simulink library "magField_reduced_lib"  (R2018b)
settings: Solver=VariableStepAuto  StartTime=0.0  StopTime=10.0  RelTol=1e-3
undefined symbols (not defined in the file or in its folder): fswParams, magField_lib, simParams
libraries: simulink_extras x2, aerolibgravity2 x1
settings Model: Creator=colem  LastModifiedBy=colem

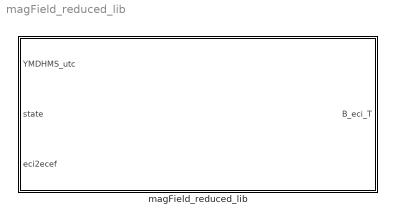
== system magField_reduced_lib ==
  magField_reduced_lib : Subsystem  AncestorBlock=magField_lib/magField_lib

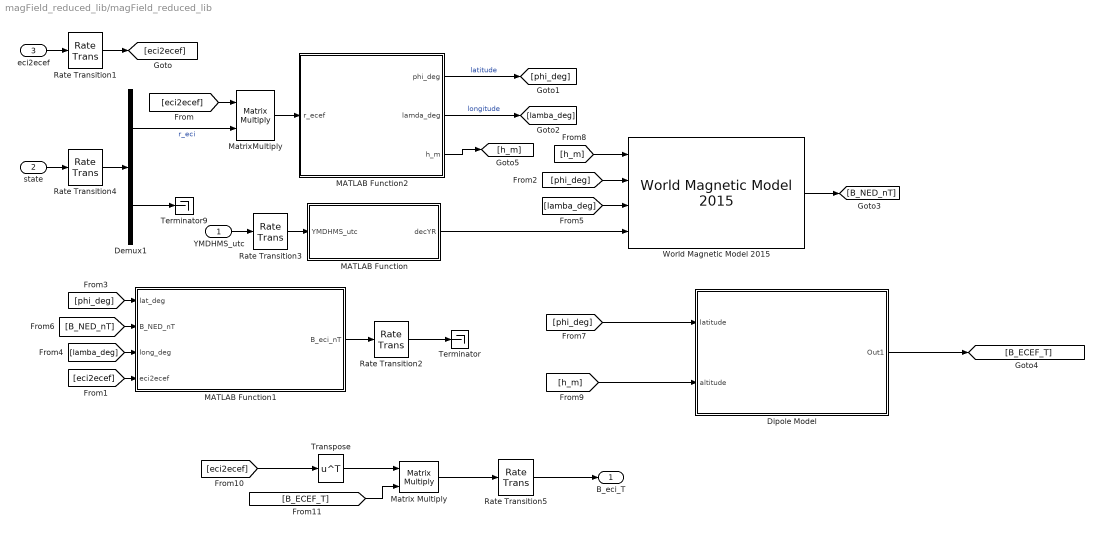
== system magField_reduced_lib/magField_reduced_lib ==
  YMDHMS_utc : Inport
  state : Inport  Port=2
  eci2ecef : Inport  Port=3
  Demux1 : Demux  Outputs=[3 10]
  Dipole Model : Subsystem
  MATLAB Function : MATLAB Function  TreatAsAtomicUnit=on
  MATLAB Function1 : MATLAB Function  TreatAsAtomicUnit=on
  MATLAB Function2 : MATLAB Function  TreatAsAtomicUnit=on
  Matrix Multiply : Product  Multiplication=Matrix(*)
  MatrixMultiply : Product  Multiplication=Matrix(*)
  Rate Transition1 : RateTransition  OutPortSampleTime=simParams.magField.sample_time_s
  Rate Transition2 : RateTransition
  Rate Transition3 : RateTransition  OutPortSampleTime=simParams.magField.sample_time_s
  Rate Transition4 : RateTransition  OutPortSampleTime=simParams.magField.sample_time_s
  Rate Transition5 : RateTransition
  Terminator : Terminator
  Terminator9 : Terminator
  Transpose : Math  Operator=transpose  SaturateOnIntegerOverflow=on
  World Magnetic Model 2015 : aerolibgravity2/World Magnetic Model 2015  units=Metric (MKS)  time_in=on  month=January  day=1  year=2015  action=None  h_out=off  dec_out=off  inc_out=off  ti_out=off
      settings: SourceProductName=Aerospace Blockset  SourceProductBaseCode=AE
  B_eci_T : Outport
  wires:
  MATLAB Function/1(decYR) -> World Magnetic Model 2015/4
  MATLAB Function1/1(B_eci_nT) -> Rate Transition2/1
  YMDHMS_utc/1 -> Rate Transition3/1
  Demux1/2 -> Terminator9/1
  Demux1/1 -> MatrixMultiply/2  "r_eci"
  state/1 -> Rate Transition4/1
  MatrixMultiply/1 -> MATLAB Function2/1(r_ecef)
  eci2ecef/1 -> Rate Transition1/1
  [eci2ecef] -> MatrixMultiply/1
  [eci2ecef] -> MATLAB Function1/4(eci2ecef)
  Rate Transition4/1 -> Demux1/1
  Rate Transition1/1 -> [eci2ecef]
  Rate Transition2/1 -> Terminator/1
  Rate Transition3/1 -> MATLAB Function/1(YMDHMS_utc)
  [phi_deg] -> World Magnetic Model 2015/2
  [phi_deg] -> MATLAB Function1/1(lat_deg)
  MATLAB Function2/2(lamda_deg) -> [lamba_deg]  "longitude"
  [lamba_deg] -> World Magnetic Model 2015/3
  World Magnetic Model 2015/1 -> [B_NED_nT]
  [B_NED_nT] -> MATLAB Function1/2(B_NED_nT)
  [lamba_deg] -> MATLAB Function1/3(long_deg)
  MATLAB Function2/1(phi_deg) -> [phi_deg]  "latitude"
  Dipole Model/1(Out1) -> [B_ECEF_T]
  [phi_deg] -> Dipole Model/1(latitude)
  MATLAB Function2/3(h_m) -> [h_m]
  [h_m] -> World Magnetic Model 2015/1
  [h_m] -> Dipole Model/2(altitude)
  [eci2ecef] -> Transpose/1
  Transpose/1 -> Matrix Multiply/1
  [B_ECEF_T] -> Matrix Multiply/2
  Rate Transition5/1 -> B_eci_T/1
  Matrix Multiply/1 -> Rate Transition5/1

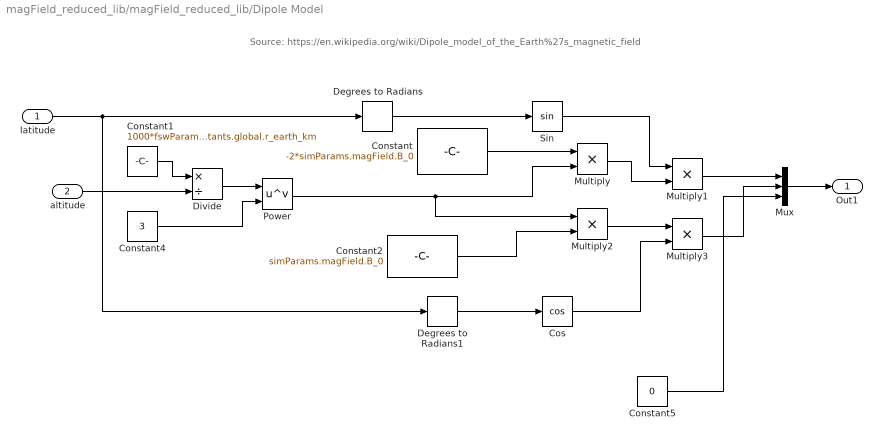
== system magField_reduced_lib/magField_reduced_lib/Dipole Model ==
  note: Source: https://en.wikipedia.org/wiki/Dipole_model_of_the_Earth%27s_magnetic_field
  latitude : Inport
  altitude : Inport  Port=2
  Constant : Constant  Value=-2*simParams.magField.B_0
  Constant1 : Constant  Value=1000*fswParams.constants.global.r_earth_km
  Constant2 : Constant  Value=simParams.magField.B_0
  Constant4 : Constant  Value=3
  Constant5 : Constant  Value=0
  Cos : Trigonometry  Operator=cos
  Degrees to Radians : simulink_extras/Transformations/Degrees to Radians
  Degrees to Radians1 : simulink_extras/Transformations/Degrees to Radians
  Divide : Product  Inputs=*/
  Multiply{,1..3} (4 alike) : Product
  Mux : Mux  Inputs=3
  Power : Math  Operator=pow  SaturateOnIntegerOverflow=on
  Sin : Trigonometry
  Out1 : Outport
  wires:
  Constant5/1 -> Mux/3
  altitude/1 -> Divide/2
  Constant1/1 -> Divide/1
  Cos/1 -> Multiply3/2
  Divide/1 -> Power/1
  Degrees to Radians1/1 -> Cos/1
  Degrees to Radians/1 -> Sin/1
  Sin/1 -> Multiply1/1
  Multiply1/1 -> Mux/1
  Constant4/1 -> Power/2
  Power/1 -> Multiply2/1, Multiply/2
  Multiply/1 -> Multiply1/2
  Constant/1 -> Multiply/1
  Constant2/1 -> Multiply2/2
  Multiply2/1 -> Multiply3/1
  latitude/1 -> Degrees to Radians1/1, Degrees to Radians/1
  Multiply3/1 -> Mux/2
  Mux/1 -> Out1/1

== matlab function magField_reduced_lib/MATLAB Function1 ==
  data: lat_deg input; B_NED_nT input; B_eci_nT output; long_deg input; eci2ecef input
function B_eci_nT = ned2eci(lat_deg,B_NED_nT,long_deg,eci2ecef)
%NED to ECEF
DCMef=zeros(3);
%source:https://www.mathworks.com/help/aeroblks/directioncosinematrixeceftoned.html
DCMef=[-sind(lat_deg)*cosd(long_deg) -sind(lat_deg)*sind(long_deg) cosd(lat_deg);...
    -sind(long_deg) cosd(long_deg) 0;...
    -cosd(lat_deg)*cosd(long_deg) -cosd(lat_deg)*sind(long_deg) -sind(lat_deg)];

B_ecef=transpose(DCMef)*B_NED_nT;

%ECEF to ECI using transformation matrix from time lib
B_eci_nT=transpose(eci2ecef)*B_ecef; %eci2ecef transformation matrix given by time_lib
end

== matlab function magField_reduced_lib/MATLAB Function ==
  data: YMDHMS_utc input; decYR output
%function converts YMDHMS array to decimal years
function decYR = decyr(YMDHMS_utc)
year=YMDHMS_utc(1)+1970; %1970 epoch
month=YMDHMS_utc(2);
day=YMDHMS_utc(3);
hour=YMDHMS_utc(4);
min=YMDHMS_utc(5);
sec=YMDHMS_utc(6);

janD=31;
marchD=31;
aprilD=30;
mayD=31;
juneD=30;
julyD=31;
augD=31;
septD=30;
octD=31;
novD=30;



if mod(year,4)==0 %leap year
    daysT=366; %total days in year
    fedD=29;
else
    daysT=365;
    fedD=28;
end
    
if month == 1
    daysS= day; %days so far
elseif month ==2
    daysS=janD+day;
elseif month ==3
    daysS=janD+fedD+day;
elseif month==4
    daysS=janD+fedD+marchD+day;
elseif month==5
    daysS=janD+fedD+marchD+aprilD+day;
elseif month==6
    daysS=janD+fedD+marchD+aprilD+mayD+day;
elseif month==7
    daysS=janD+fedD+marchD+aprilD+mayD+juneD+day;
elseif month==8
    daysS=janD+fedD+marchD+aprilD+mayD+juneD+julyD+day;
elseif month==9
    daysS=janD+fedD+marchD+aprilD+mayD+juneD+julyD+augD+day;
elseif month==10
    daysS=janD+fedD+marchD+aprilD+mayD+juneD+julyD+augD+septD+day;
elseif month==11
    daysS=janD+fedD+marchD+aprilD+mayD+juneD+julyD+augD+septD+octD+day;
else %dec
    daysS=janD+fedD+marchD+aprilD+mayD+juneD+julyD+augD+septD+octD+novD+day;
end

%add time of day component
daysS=daysS+hour/24+min/1440+sec/86400;
decYR=year+daysS/daysT;
end

== matlab function magField_reduced_lib/MATLAB Function2 ==
  data: r_ecef input; phi_deg output; lamda_deg output; h_m output
function [phi_deg,lamda_deg,h_m] = ECEF_to_LatLon2(r_ecef)

%Author: Devan, Ivan
    %ECEF_TO_LA Summary of this function goes here
    %Transforms from a given ECEF radial vector to the latitude (phi) and
    %longitude vectors (lamba)(he). This uses Algorithm 12 (pg 173)

    tol = .0001; %Tolerance of the iterations
    
    
    % Defind the IJK radial components  
    rI = r_ecef(1);
    rJ = r_ecef(2);
    rK = r_ecef(3);
    
    %Define radius and eccentricity of earth (note: not e of earths orbit)
    re =  6378.1363;
    e = 0.081819221456;

    %This is the magditude of the satellites distance   
    r_dsat = sqrt(rI^2 + rJ^2);

    %Calculate the sin(a) and cos(a)       
    sina = rJ/r_dsat;
    cosa = rI/r_dsat;
    
    %Correct for quadrant error 
    %a = quadCheck(cosa,sina);
    a=atan2(sina,cosa); %This is better and you don't need to learn angles. 
    
    %once corrected lambda is simply the angle alpha (a)
    lamda_deg = a*180/pi;
    
    end_flag = 0;
    
    %Now solve iteratively for phi    
    phi_old = atan2(rK,r_dsat);
    
    %Calculate C for first iteration
    C = re/sqrt(1 - (e^2)*(sin(phi_old)^2) );
    
    %tanphid = (rK + C*(e^2)*sin(phi_old))/r_dsat;
    phi_gd = atan2(rK + C*(e^2)*sin(phi_old),r_dsat);
    %print = phi_gd*180/pi  %in case you want to check
    
    %this will break us out of the loop  
    if abs(phi_gd - phi_old) < tol
        end_flag = 1;
  
    else
        phi_old = phi_gd;
        end_flag = 0;
    end
    
    count = 0;
    
    while (end_flag == 0)
        C = re/sqrt(1 - (e^2)*(sin(phi_old)^2) );
        %tanphid = (rK + C*(e^2)*sin(phi_old))/r_dsat;
        %phi_gd = atan(tanphid);
        phi_gd = atan2(rK + C*(e^2)*sin(phi_old),r_dsat);
        
        if abs(phi_gd - phi_old) < tol
            end_flag = 1;
        else
            phi_old = phi_gd;
            end_flag = 0;
        end
        count = count + 1;
        
        if count >= 100
            end_flag = 0; 
        end
    end
    
    C = re/sqrt(1 - (e^2)*(sin(phi_gd)^2) );
    phi_deg = phi_gd*180/pi;
    Se = C*(1 - e^2);
    if phi_deg < 1
        h_m = rK/(sin(phi_gd)) - Se;
%         print(' < 1 case')
    else
        h_m = r_dsat/(cosd(phi_deg)) - C;
%         print(' Regular Case ')
    end
    
    h_m=h_m*1000;
end
